simulink model "Ramon24210589P1"  (R2026a)
settings: Solver=VariableStepAuto  StopTime=50
libraries: fl_lib x8, nesl_utility x3, slpidlib x1, simulink x1, ee_lib x1
settings Model: LastModifiedBy=HP
settings SolverCC: AlgebraicLoopSolver=LineSearch
settings DataIOCC: TimeSaveName=t
settings DebuggingCC: ArtificialAlgebraicLoopMsg=none  MaxConsecutiveZCsMsg=none  OperatingPointInterfaceChecksumMismatchMsg=none
settings SimscapeCC: SimscapeNominalValues="[{\"value\":\"1\",\"unit\":\"A\"},{\"value\":\"1\",\"unit\":\"bar\"},{\"value\":\"1\",\"unit\":\"cm^2\"},{\"value\":\"1\",\"unit\":\"cm^3/s\"},{\"value\":\"1\",\"unit\":\"kJ/kg\"},{\"value\":\"1\",\"unit\":\"kW\"},{\"value\":\"1\",\"unit\":\"l\"},{\"value\":\"1\",\"unit\":\"N\"},{\"value\":\"1\",\"unit\":\"N*m\"},{\"value\":\"1\",\"unit\":\"V\"}]"  SimscapeLogType=none  SimscapeLogDataHistory=5000.0

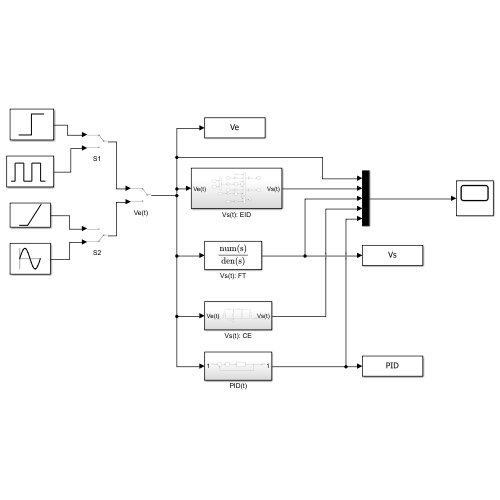
[thumbnail: Simulink's stored preview of the top-level diagram]
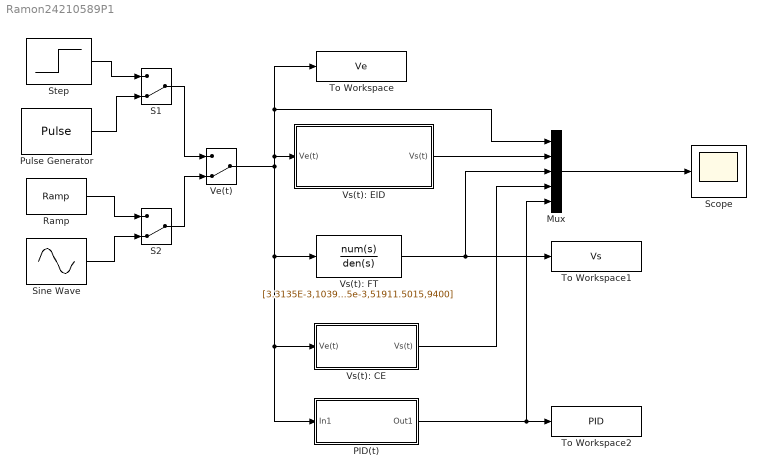
== system Ramon24210589P1 ==
  Mux : Mux  Inputs=5
  PID(t) : Subsystem
  Pulse Generator : DiscretePulseGenerator  PulseType=Time based  Period=10  PulseWidth=10  PhaseDelay=1
  Ramp : simulink/Sources/Ramp  slope=1/10  start=0  InitialOutput=0
  S1 : ManualSwitch  CurrentSetting=0
  S2 : ManualSwitch  CurrentSetting=0
  Scope : Scope
      settings: ActiveDisplayYMinimum=-0.36262  ActiveDisplayYMaximum=1.26358
  Sine Wave : Sin  Frequency=pi/2
  Step : Step  Time=0  InitialValue=1  SampleTime=0
  To Workspace : ToWorkspace  VariableName=Ve  SampleTime=-1
  To Workspace1 : ToWorkspace  VariableName=Vs  SampleTime=-1
  To Workspace2 : ToWorkspace  VariableName=PID  SampleTime=-1
  Ve(t) : ManualSwitch  CurrentSetting=0
  Vs(t): CE : Subsystem
  Vs(t): EID : Subsystem
  Vs(t): FT : TransferFcn  Numerator=[3.3135E-3,10392.3015,4700]  Denominator=[9.9405e-3,51911.5015,9400]
  wires:
  Mux/1 -> Scope/1
  Vs(t): EID/1(Vs(t)) -> Mux/2
  Step/1 -> S1/1
  Pulse Generator/1 -> S1/2
  Ramp/1 -> S2/1
  Sine Wave/1 -> S2/2
  S2/1 -> Ve(t)/2
  S1/1 -> Ve(t)/1
  Vs(t): FT/1 -> To Workspace1/1, Mux/3
  Vs(t): CE/1(Vs(t)) -> Mux/4
  PID(t)/1(Out1) -> To Workspace2/1, Mux/5
  Ve(t)/1 -> To Workspace/1, Mux/1, Vs(t): EID/1(Ve(t)), PID(t)/1(In1), Vs(t): CE/1(Ve(t)), Vs(t): FT/1

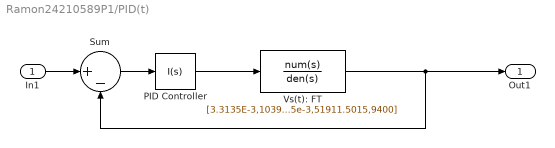
== system Ramon24210589P1/PID(t) ==
  In1 : Inport
  PID Controller : slpidlib/PID Controller  Controller=I  Form=Parallel  TimeDomain=Continuous-time  UseExternalTs=off  SampleTime=-1  IntegratorMethod=Forward Euler  FilterMethod=Forward Euler  ControllerParametersSource=internal  P=0  I=379.856619065551  UseKiTs=off  D=0  UseExternalDerivativeSource=off  N=100  UseFilter=on  TunerSelectOption=Transfer Function Based (PID Tuner App)  InitialConditionSource=internal  InitialConditionForIntegrator=0  InitialConditionForFilter=0  DifferentiatorICPrevScaledInput=0  ExternalReset=none  TrackingMode=off  Kt=1  LimitOutput=off  SatLimitsSource=internal  UpperSaturationLimit=inf  LowerSaturationLimit=-inf  LinearizeAsGain=on  AntiWindupMode=none  Kb=1  LimitIntegrator=off  UpperIntegratorSaturationLimit=inf  LowerIntegratorSaturationLimit=-inf  POutMin=[]  POutMax=[]  IOutMin=[]  IOutMax=[]  DOutMin=[]  DOutMax=[]  NOutMin=[]  NOutMax=[]  SumOutMin=[]  SumOutMax=[]  SaturationOutMin=[]  SaturationOutMax=[]  PParamMin=[]  PParamMax=[]  IParamMin=[]  IParamMax=[]  DParamMin=[]  DParamMax=[]  NParamMin=[]  NParamMax=[]  KbParamMin=[]  KbParamMax=[]  KtParamMin=[]  KtParamMax=[]  KbOutMin=[]  KbOutMax=[]  KtOutMin=[]  KtOutMax=[]  IntegratorOutMin=[]  IntegratorOutMax=[]  FilterOutMin=[]  FilterOutMax=[]  SumI1OutMin=[]  SumI1OutMax=[]  SumI2OutMin=[]  SumI2OutMax=[]  SumI3OutMin=[]  SumI3OutMax=[]  SumI4OutMin=[]  SumI4OutMax=[]  SumDOutMin=[]  SumDOutMax=[]  DifferentiatorOutMin=[]  DifferentiatorOutMax=[]  FilterDiffOutCoefMin=[]  FilterDiffOutCoefMax=[]  ReciprocalOutMin=[]  ReciprocalOutMax=[]  SumDenOutMin=[]  SumDenOutMax=[]  SumNumOutMin=[]  SumNumOutMax=[]  DivideOutMin=[]  DivideOutMax=[]  UdiffTsProdOutMin=[]  UdiffTsProdOutMax=[]  NTsProdOutMin=[]  NTsProdOutMax=[]  UintegralTsProdOutMin=[]  UintegralTsProdOutMax=[]  UngainTsProdOutMin=[]  UngainTsProdOutMax=[]  ClampingZeroOutDataTypeStr=Inherit: Inherit via back propagation  ClampingZeroOutMin=[]  ClampingZeroOutMax=[]  FilterDenConstantOutDataTypeStr=Inherit: Inherit via back propagation  FilterDenConstantOutMin=[]  FilterDenConstantOutMax=[]  PCopyOutDataTypeStr=Inherit: Inherit via back propagation  PCopyOutMin=[]  PCopyOutMax=[]  NCopyOutDataTypeStr=Inherit: Inherit via back propagation  NCopyOutMin=[]  NCopyOutMax=[]  IntegratorContinuousStateAttributes=''  IntegratorStateMustResolveToSignalObject=off  IntegratorRTWStateStorageClass=Auto  FilterContinuousStateAttributes=''  FilterStateMustResolveToSignalObject=off  FilterRTWStateStorageClass=Auto  ParallelPVariant=Disabled  IdealPVariant=Disabled  IVariant=InternalParameters  DVariant=Disabled  IntegratorVariant=Continuous  SatVariant=Disabled  AWVariant=Passthrough  PCopyVariant=Disabled  TRVariant=Disabled  FdbkBlocksVariant=Forward  IdealPFdbkVariant=Disabled  SatFdbkVariant=Disabled  DerivativeFilterVariant=Disabled  NVariant=Disabled  NCopyVariant=Disabled_SignalSpec  FilterICVariant=Disabled  IntegratorICVariant=InternalICs  ExternalResetVariant=Disabled  TRSumVariant=Passthrough  SumFdbkVariant=Disabled  SumVariant=Passthrough_I  TsampFilterVariant=InternalTs  TsampNgainVariant=Passthrough  TsampIntegralVariant=Disabled_SignalSpec  ExternalSaturationOutDataTypeStr=Inherit: Same as second input  DerivativeSourceVariant=Disabled  PreIntVariant=InternalPreInt
  Sum : Sum  Inputs=|+-
  Vs(t): FT : TransferFcn  Numerator=[3.3135E-3,10392.3015,4700]  Denominator=[9.9405e-3,51911.5015,9400]
  Out1 : Outport
  wires:
  Sum/1 -> PID Controller/1
  In1/1 -> Sum/1
  PID Controller/1 -> Vs(t): FT/1
  Vs(t): FT/1 -> Sum/2, Out1/1

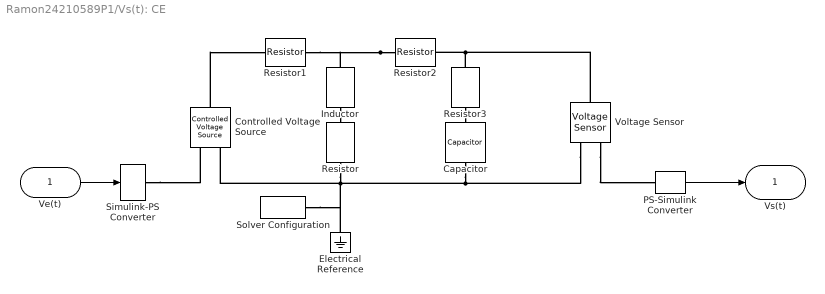
== system Ramon24210589P1/Vs(t): CE ==
  Ve(t) : Inport
  Capacitor : fl_lib/Electrical/Electrical Elements/Capacitor  c=470E-6 F  r=1e-6 Ohm  g=0 1/Ohm  i_specify=off  i_priority=None  i=0 A  i_nominal_specify=off  i_nominal_value=1  i_nominal_unit=A  v_specify=off  v_priority=None  v=0 V  v_nominal_specify=off  v_nominal_value=1  v_nominal_unit=V  vc_specify=off  vc_priority=High  vc=0 V  vc_nominal_specify=off  vc_nominal_value=1  vc_nominal_unit=V
  Controlled Voltage Source : fl_lib/Electrical/Electrical Sources/Controlled Voltage Source
  Electrical Reference : fl_lib/Electrical/Electrical Elements/Electrical Reference
  Inductor : ee_lib/Passive/Inductor  l=1.5E-3 H  enable_L_tol=0  L_tol=20  tol_distribution=1  nSigma=4  r=0 Ohm  g=1e-9 1/Ohm  enable_operating_limits=0  operating_limit_action=2  max_working_current=1 A  power_rating=1 W  i_L_specify=off  i_L_priority=High  i_L=0 A  i_L_nominal_specify=off  i_L_nominal_value=1  i_L_nominal_unit=A
  PS-Simulink Converter : nesl_utility/PS-Simulink Converter  PhysicalDomain=network_engine_domain  SubClassName=ps_output  LeftPortType=input  RightPortType=output  PseudoPeriodic=off  Frequencies=[]  VectorFormat=1-D array  Unit=inherit  AffineConversion=off
  Resistor{,1..3} (4 alike) : fl_lib/Electrical/Electrical Elements/Resistor  R=4.7E3 Ohm  i_specify=off  i_priority=None  i=0 A  i_nominal_specify=off  i_nominal_value=1  i_nominal_unit=A  v_specify=off  v_priority=None  v=0 V  v_nominal_specify=off  v_nominal_value=1  v_nominal_unit=V
  Simulink-PS Converter : nesl_utility/Simulink-PS Converter  PhysicalDomain=network_engine_domain  SubClassName=ps_input  LeftPortType=input  RightPortType=output  PseudoPeriodic=off  Frequencies=[]  NoiseDistribution=none  NoiseParameters=[]  Unit=1  AffineConversion=off  FilteringAndDerivatives=provide  SimscapeFilterOrder=1  InputFilterTimeConstant=0.001  UdotUserProvided=0
  Solver Configuration : nesl_utility/Solver Configuration  PhysicalDomain=network_engine_domain  SubClassName=solver  LeftPortType=input  RightPortType=generic  Tones=[]  Harmonics=[]  SimulateNoise=off  Profile=off  UseLocalSampling=off  EnableSwitchedLinearOptims=on  FrequencyDomain=off  UseCCode=off  RelTol=0.001  AbsTol=1e-06  MinStep=1e-09  ToWorkspace=off  RevertToSquareIcSolve=off  NumHomotopyIterations=100  PhasorMode=off  PhasorModeNumHarmonics=1  ConsistencySolver=NEWTON_FTOL  CanonicalOrdering=UNORDERED  OptimizeIntermediates=UNOPTIMIZED  IndexReductionMethod=DerivativeReplacement  DoDC=off  ResidualTolerance=1e-09  ConsistencyTolSource=GLOBAL  ConsistencyAbsTol=0.001  ConsistencyRelTol=0.001  ConsistencyTolFactor=0.001  UseLocalSolver=off  LocalSolverChoice=NE_BACKWARD_EULER_ADVANCER  ResolveIndetEquations=on  FunctionEvalNumThread=1  LocalSolverSampleTime=0.001  DoFixedCost=off  MaxNonlinIter=3  MaxModeIter=2  ComputeImpulses=off  ImpulseIterations=2  LinearAlgebra=auto  LinearAlgebraNumThread=0  EquationFormulation=NE_TIME_EF  DelaysMemoryBudget=1024  AutomaticFiltering=on  FilteringTimeConstant=0.001  PartitionStorageMethod=AS_NEEDED  PartitionMemoryBudget=1024  PartitionMethod=ROBUST  MultibodyUseLocalSolver=off  MultibodyLocalSolverChoice=ODE1  MultibodyLocalSolverSampleTime=0.001
  Voltage Sensor : fl_lib/Electrical/Electrical Sensors/Voltage Sensor
  Vs(t) : Outport
  wires:
  Ve(t)/1 -> Simulink-PS Converter/1
  PS-Simulink Converter/1 -> Vs(t)/1
  connections:
  Simulink-PS Converter/RConn1 -- Controlled Voltage Source/RConn1
  Voltage Sensor/RConn1 -- PS-Simulink Converter/LConn1
  Voltage Sensor/RConn2 -- Capacitor/RConn1 -- Resistor/RConn1 -- Electrical Reference/LConn1 -- Solver Configuration/RConn1 -- Controlled Voltage Source/RConn2
  Resistor2/LConn1 -- Inductor/LConn1 -- Resistor1/RConn1
  Controlled Voltage Source/LConn1 -- Resistor1/LConn1
  Inductor/RConn1 -- Resistor/LConn1
  Resistor3/LConn1 -- Voltage Sensor/LConn1 -- Resistor2/RConn1
  Resistor3/RConn1 -- Capacitor/LConn1

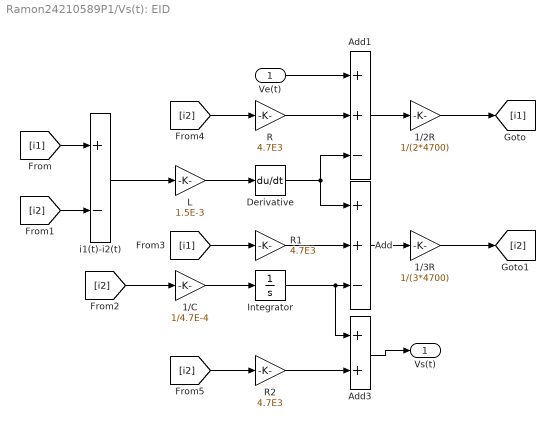
== system Ramon24210589P1/Vs(t): EID ==
  Ve(t) : Inport
  1/2R : Gain  Gain=1/(2*4700)
  1/3R : Gain  Gain=1/(3*4700)
  1/C : Gain  Gain=1/4.7E-4
  Add : Sum  Inputs=++-
  Add1 : Sum  Inputs=++-
  Add3 : Sum
  Derivative : Derivative
  Integrator : Integrator
  L : Gain  Gain=1.5E-3
  R : Gain  Gain=4.7E3
  R1 : Gain  Gain=4.7E3
  R2 : Gain  Gain=4.7E3
  i1(t)-i2(t) : Sum  Inputs=+-
  Vs(t) : Outport
  wires:
  1/2R/1 -> [i1]
  1/3R/1 -> [i2]
  Add/1 -> 1/3R/1
  Add1/1 -> 1/2R/1
  Derivative/1 -> Add/1, Add1/3
  L/1 -> Derivative/1
  i1(t)-i2(t)/1 -> L/1
  Ve(t)/1 -> Add1/1
  R/1 -> Add1/2
  Integrator/1 -> Add3/1, Add/3
  1/C/1 -> Integrator/1
  [i1] -> i1(t)-i2(t)/1
  [i2] -> i1(t)-i2(t)/2
  [i2] -> 1/C/1
  R1/1 -> Add/2
  [i1] -> R1/1
  [i2] -> R/1
  Add3/1 -> Vs(t)/1
  R2/1 -> Add3/2
  [i2] -> R2/1
